simulink model "TAULab2"  (R2014b)
settings: Solver=ode45  StartTime=0.0  StopTime=10.0  RelTol=1e-3
settings Model: Creator=kiril_000  LastModifiedBy=kiril_000

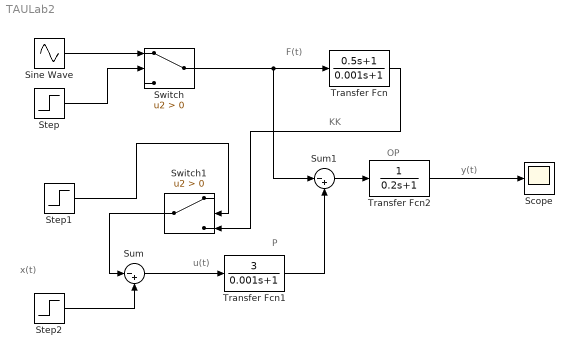
== system TAULab2 ==
  note: KK
  note: OP
  note: P
  note: u(t)
  note: F(t)
  note: y(t)
  note: x(t)
  Scope : Scope
      settings: YMin=-1  YMax=1
  Sine Wave : Sin  Frequency=10  SampleTime=0
  Step : Step  SampleTime=2
  Step1 : Step  SampleTime=4
  Step2 : Step  SampleTime=0
  Sum : Sum  Inputs=|-+
  Sum1 : Sum  Inputs=|-+
  Switch : Switch  Criteria=u2 > Threshold
  Switch1 : Switch  Criteria=u2 > Threshold
  Transfer Fcn : TransferFcn  Numerator=[0.5 1]  Denominator=[0.001 1]
  Transfer Fcn1 : TransferFcn  Numerator=[3]  Denominator=[0.001 1]
  Transfer Fcn2 : TransferFcn  Denominator=[0.2 1]
  wires:
  Sine Wave/1 -> Switch/1
  Step/1 -> Switch/2
  Switch/1 -> Sum1/1, Transfer Fcn/1
  Transfer Fcn/1 -> Switch1/3
  Step1/1 -> Switch1/2
  Switch1/1 -> Sum/1
  Step2/1 -> Sum/2
  Sum/1 -> Transfer Fcn1/1
  Transfer Fcn1/1 -> Sum1/2
  Sum1/1 -> Transfer Fcn2/1
  Transfer Fcn2/1 -> Scope/1
